simulink model "Simulink_Lab2_2"  (R2015a)
settings: Solver=ode5  StartTime=0.0  StopTime=10.0  FixedStep=0.01  RelTol=1e-3
values from neighbouring files (symbols this model uses):
  C = 100    [Lab_2.m]
  K = 1000    [Lab_2.m]
  m = 10    [Lab_2.m]
settings Model: Creator=009768408  LastModifiedBy=009768408
settings DataIOCC: SaveOutput=off  SaveTime=off

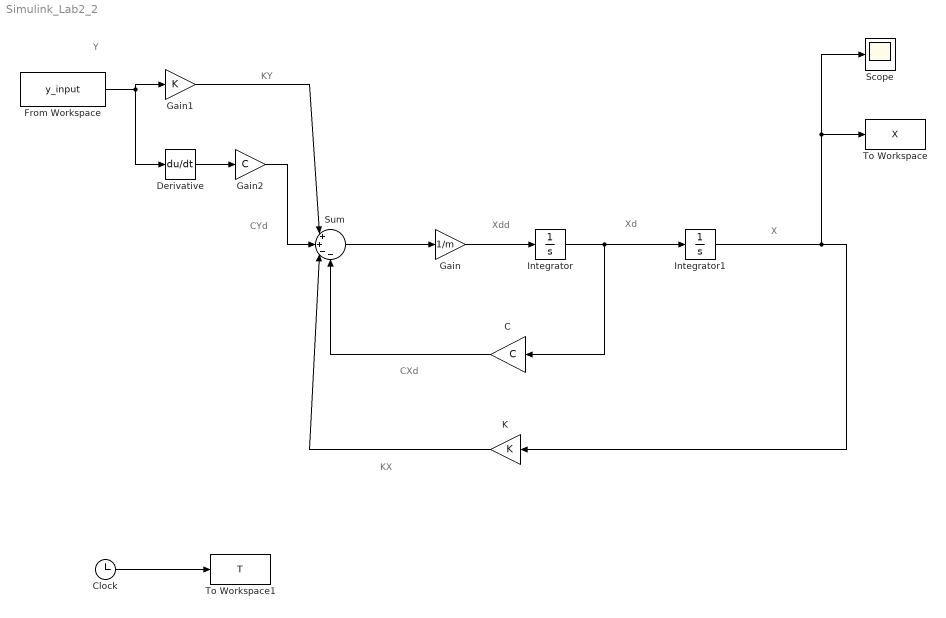
== system Simulink_Lab2_2 ==
  note: Y
  note: CYd
  note: KY
  note: CXd
  note: KX
  note: X
  note: Xd
  note: Xdd
  C : Gain  Gain=C
  Clock : Clock
  Derivative : Derivative
  From Workspace : FromWorkspace  VariableName=y_input  SampleTime=0
  Gain : Gain  Gain=1/m
  Gain1 : Gain  Gain=K
  Gain2 : Gain  Gain=C
  Integrator : Integrator
  Integrator1 : Integrator
  K : Gain  Gain=K
  Scope : Scope
  Sum : Sum  Inputs=|++--
  To Workspace : ToWorkspace  VariableName=X  SampleTime=-1
  To Workspace1 : ToWorkspace  VariableName=T  SampleTime=-1
  wires:
  Sum/1 -> Gain/1
  Integrator1/1 -> Scope/1, To Workspace/1, K/1
  K/1 -> Sum/3
  Integrator/1 -> C/1, Integrator1/1
  Gain/1 -> Integrator/1
  C/1 -> Sum/4
  From Workspace/1 -> Gain1/1, Derivative/1
  Derivative/1 -> Gain2/1
  Gain1/1 -> Sum/1
  Gain2/1 -> Sum/2
  Clock/1 -> To Workspace1/1
